simulink model "QCS"  (R2020b)
settings: Solver=ode3  StartTime=0.0  StopTime=30  FixedStep=Ts  RelTol=1e-3
undefined symbols (not defined in the file): Ts
libraries: SignalEditorBlockLib x2, sharedtransform x1, uavutilslib x1
settings Model: Creator=dbell44  LastModifiedBy=dbell44
settings DebuggingCC: BusObjectLabelMismatch=none

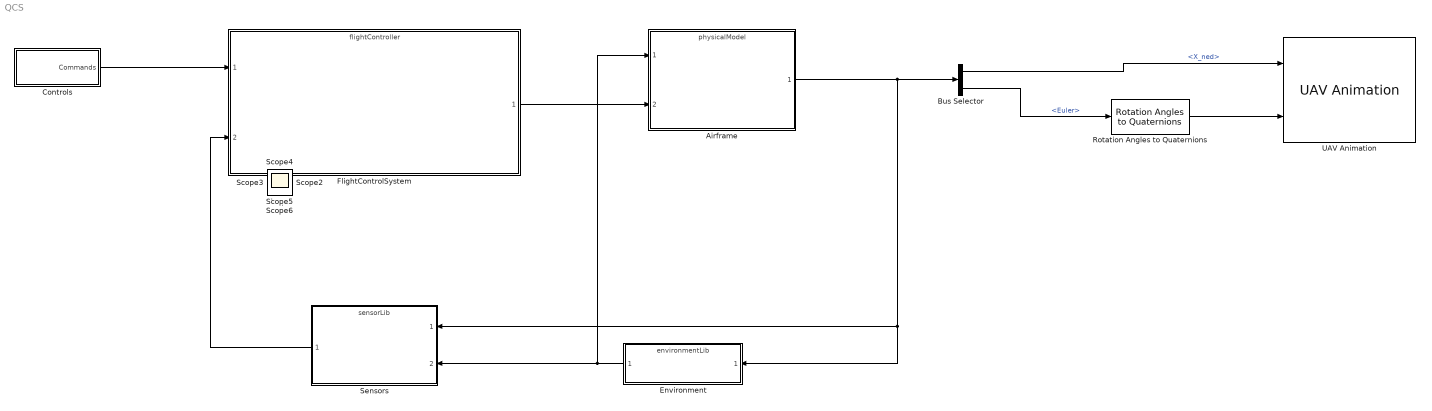
== system QCS ==
  Airframe : ModelReference  ModelNameDialog=physicalModel.slx  SimulationMode=Normal  ModelReferenceVersion=2.8
  Bus Selector : BusSelector  OutputSignals=X_ned,Euler
  Controls : Subsystem
  Environment : ModelReference  ModelNameDialog=environmentLib.slx  SimulationMode=Normal  ModelReferenceVersion=2.1
  FlightControlSystem : ModelReference  ModelNameDialog=flightController.slx  SimulationMode=Normal  ModelReferenceVersion=1.7
  Rotation Angles to Quaternions : sharedtransform/Rotation Angles to Quaternions  rotationOrder=XYZ  aMode=aMode
      settings: SourceProductBaseCode=AE,PW,MT,UV,VE,VP
  Sensors : ModelReference  ModelNameDialog=sensorLib.slx  SimulationMode=Normal  ModelReferenceVersion=1.43
  UAV Animation : uavutilslib/UAV Animation  UAVType=Multirotor  UAVSize=1  InertialZDirection=Down  SampleTime=-1
      settings: SourceProductBaseCode=UV
  Scope{,1..6} (7 alike) : Scope
  wires:
  Environment/1 -> Airframe/1, Sensors/2
  Airframe/1 -> Sensors/1, Environment/1, Bus Selector/1
  Controls/1(Commands) -> FlightControlSystem/1
  FlightControlSystem/1 -> Airframe/2
  Rotation Angles to Quaternions/1 -> UAV Animation/2
  Bus Selector/1 -> UAV Animation/1  "<X_ned>"
  Bus Selector/2 -> Rotation Angles to Quaternions/1  "<Euler>"
  Sensors/1 -> FlightControlSystem/2

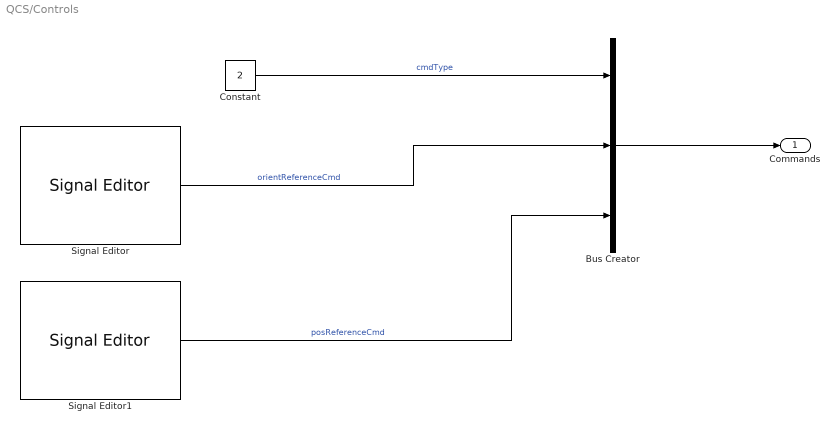
== system QCS/Controls ==
  Bus Creator : BusCreator  Inputs=3  OutDataTypeStr=Bus: CommandBus
      settings: InheritFromInputs=off
  Constant : Constant  Value=2  OutDataTypeStr=uint8
  Signal Editor : SignalEditorBlockLib/Signal Editor  FileName=orientRefHover.mat  ActiveScenario=Circle  ActiveSignal=orientReferenceCmd  IsBus=on  OutputBusObjectStr=Bus: Orientation_Ref  SampleTime=0  Interpolate=off  ZeroCross=off  OutputAfterFinalValue=Setting to zero  Unit=inherit  PreserveSignalName=on
  Signal Editor1 : SignalEditorBlockLib/Signal Editor  FileName=posRefHover.mat  ActiveScenario=FlyCircle  ActiveSignal=posReferenceCmd  IsBus=on  OutputBusObjectStr=Bus: Position_Ref  SampleTime=Ts  Interpolate=off  ZeroCross=off  OutputAfterFinalValue=Setting to zero  Unit=inherit  PreserveSignalName=on
  Commands : Outport  OutDataTypeStr=Bus: CommandBus
  wires:
  Constant/1 -> Bus Creator/1  "cmdType"
  Signal Editor/1 -> Bus Creator/2  "orientReferenceCmd"
  Signal Editor1/1 -> Bus Creator/3  "posReferenceCmd"
  Bus Creator/1 -> Commands/1
